simulink model "ammclib_gflib_limit_s32k14x"  (Simulink 9.0)
settings: Solver=FixedStepDiscrete  StartTime=0.0  StopTime=5  FixedStep=0.001  RelTol=1e-3  EnableMultiTasking=on
InitFcn:
  | mbd_s32k_consistency_checks(bdroot(gcs));
undefined symbols (not defined in the file or in its folder): LQFP
libraries: ammclib_bam_s32k14x x23, simulink x16, mbd_s32k1xx_ec_toolbox x2
Description:
  | This model tests the AMMCLIB GFLIB LIMIT blocks
  | 
  | Validation:
  | - Run the model in Simulation and check the results
  | - Open Freemaster (ammclib_gflib_limit_s32k14x.pmp) and compare the HW results against the Simulated ones
CloseFcn:
  | clear all;
settings Model: Creator=NXP MBDT Team  LastModifiedBy=nxf35172
settings DataIOCC: ExternalInput=off  InitialState=off  LimitDataPoints=on  SaveOutput=off  SignalLogging=off  SaveTime=off
settings OptimizationCC: DefaultParameterBehavior=Inlined  LifeSpan=1
settings DebuggingCC: SolverPrmCheckMsg=warning  InheritedTsInSrcMsg=none  SingleTaskRateTransMsg=error  IntegerOverflowMsg=none  ParameterPrecisionLossMsg=none  UnconnectedInputMsg=error  UnconnectedOutputMsg=error  UnconnectedLineMsg=error  AllowSymbolicDim=off  UnknownTsInhSupMsg=error  StateNameClashWarn=warning
settings HardwareCC: ProdLargestAtomicInteger=Long  ProdLargestAtomicFloat=Double  ProdEndianess=LittleEndian  ProdHWDeviceType=ARM Compatible->ARM Cortex
settings SFSimCC: MATLABDynamicMemAlloc=off
settings RTWCC: SystemTargetFile=mbd_s32k.tlc  MakeCommand=mbd_s32k_make_rtw COPY_MDLREF_INCLUDES=0  TemplateMakefile=mbd_s32k.tmf  Description=Model Based Design Toolbox S32K14x Code Generation Target
settings CodeAppCC: IgnoreCustomStorageClasses=off
settings STFCustomTargetCC: CombineOutputUpdateFcns=on  ERTCustomFileBanners=on  SupportContinuousTime=off  SupportNonInlinedSFcns=off  RemoveResetFunc=on  MATLABClassNameForMDSCustomization=Simulink.SoftwareTarget.ERTCustomization  GRTInterface=off  SystemTargetFile=mbd_s32k14.tlc
settings ERTTargetCC: MultiwordLength=2048  ParMdlRefBuildCompliant=off  CompOptLevelCompliant=off  ConcurrentExecutionCompliant=off  ModelStepFunctionPrototypeControlCompliant=off  CPPClassGenCompliant=off  UseToolchainInfoCompliant=off  InlinedParameterPlacement=NonHierarchical  ERTCustomFileTemplate=example_file_process.tlc  ConvertIfToSwitch=off  SuppressUnreachableDefaultCases=off

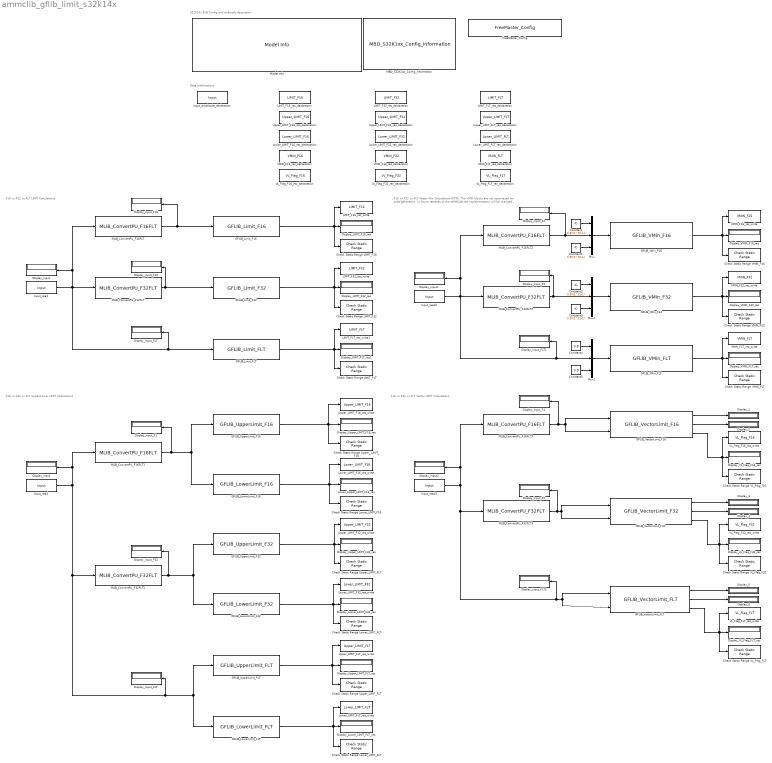
== system ammclib_gflib_limit_s32k14x ==
  note: S32K14x EVB Config and example description
  note: Data Initializations
  note: F16 vs F32 vs FLT LIMIT Calculations
  note: F16 vs F32 vs FLT Upper/Lower LIMIT Calculations
  note: F16 vs F32 vs FLT Vector Min Calculations
      | NOTE: The VMIN blocks are not optimiezed for code-generation. In future releases of the AMMCLIB the implementation will be changed
  note: F16 vs F32 vs FLT Vector LIMIT Calculations
  "Check Static Range LIMIT_F16 " : simulink/Model Verification/Check  Static Range  Description=-0.5*(2^15-1)-1 <= u <= 0.5*(2^15-1)+1  max=0.5*(2^15-1)+1  max_included=on  min=-0.5*(2^15-1)-1  min_included=on  enabled=on  stopWhenAssertionFail=on  export=off  icon=graphic
      settings: SourceProductName=Simulink  SourceProductBaseCode=SL
  Check Static Range LIMIT_F32 : simulink/Model Verification/Check  Static Range  Description=-0.5*(2^31-1)-1 <= u <= 0.5*(2^31-1)+1  max=0.5*(2^31-1)+1  max_included=on  min=-0.5*(2^31-1)-1  min_included=on  enabled=on  stopWhenAssertionFail=on  export=off  icon=graphic
      settings: SourceProductName=Simulink  SourceProductBaseCode=SL
  Check Static Range LIMIT_FLT : simulink/Model Verification/Check  Static Range  Description=-0.51 <= u <= 0.51  max=0.51  max_included=on  min=-0.51  min_included=on  enabled=on  stopWhenAssertionFail=on  export=off  icon=graphic
      settings: SourceProductName=Simulink  SourceProductBaseCode=SL
  Check Static Range Lower_LIMIT_F16 : simulink/Model Verification/Check  Static Range  Description=-0.5*(2^15-1)-1 <= u <= (2^15-1)  max=(2^15-1)  max_included=on  min=-0.5*(2^15-1)-1  min_included=on  enabled=on  stopWhenAssertionFail=on  export=off  icon=graphic
      settings: SourceProductName=Simulink  SourceProductBaseCode=SL
  Check Static Range Lower_LIMIT_FLT : simulink/Model Verification/Check  Static Range  Description=-0.5*(2^31-1)-1 <= u <= (2^31-1)  max=(2^31-1)  max_included=on  min=-0.5*(2^31-1)-1  min_included=on  enabled=on  stopWhenAssertionFail=on  export=off  icon=graphic
      settings: SourceProductName=Simulink  SourceProductBaseCode=SL
  "Check Static Range Lower_LIMIT_FLT  " : simulink/Model Verification/Check  Static Range  Description=-0.5 <= u <= 1  max=1  max_included=on  min=-0.5  min_included=on  enabled=on  stopWhenAssertionFail=on  export=off  icon=graphic
      settings: SourceProductName=Simulink  SourceProductBaseCode=SL
  "Check Static Range Upper_ LIMIT_F16 " : simulink/Model Verification/Check  Static Range  Description=-(2^15-1) <= u <= 0.5*(2^15-1)+1  max=0.5*(2^15-1)+1  max_included=on  min=-(2^15-1)  min_included=on  enabled=on  stopWhenAssertionFail=on  export=off  icon=graphic
      settings: SourceProductName=Simulink  SourceProductBaseCode=SL
  Check Static Range Upper_LIMIT_FLT : simulink/Model Verification/Check  Static Range  Description=-(2^31-1) <= u <= 0.5*(2^31-1)+1  max=0.5*(2^31-1)+1  max_included=on  min=-(2^31-1)  min_included=on  enabled=on  stopWhenAssertionFail=on  export=off  icon=graphic
      settings: SourceProductName=Simulink  SourceProductBaseCode=SL
  "Check Static Range Upper_LIMIT_FLT " : simulink/Model Verification/Check  Static Range  Description=-1 <= u <= 0.51  max=0.51  max_included=on  min=-1  min_included=on  enabled=on  stopWhenAssertionFail=on  export=off  icon=graphic
      settings: SourceProductName=Simulink  SourceProductBaseCode=SL
  Check Static Range VL_Flag_F32 : simulink/Model Verification/Check  Static Range  Description=0 <= u <= 1  max=1  max_included=on  min=0  min_included=on  enabled=on  stopWhenAssertionFail=on  export=off  icon=graphic
      settings: SourceProductName=Simulink  SourceProductBaseCode=SL
  Check Static Range VL_Flag_FLT : simulink/Model Verification/Check  Static Range  Description=0 <= u <= 1  max=1  max_included=on  min=0  min_included=on  enabled=on  stopWhenAssertionFail=on  export=off  icon=graphic
      settings: SourceProductName=Simulink  SourceProductBaseCode=SL
  Check Static Range VL_Flag_f16 : simulink/Model Verification/Check  Static Range  Description=0 <= u <= 1  max=1  max_included=on  min=0  min_included=on  enabled=on  stopWhenAssertionFail=on  export=off  icon=graphic
      settings: SourceProductName=Simulink  SourceProductBaseCode=SL
  Check Static Range VMIN_F16 : simulink/Model Verification/Check  Static Range  Description=0 <= u <= 2  max=2  max_included=on  min=0  min_included=on  enabled=on  stopWhenAssertionFail=on  export=off  icon=graphic
      settings: SourceProductName=Simulink  SourceProductBaseCode=SL
  Check Static Range VMIN_F32 : simulink/Model Verification/Check  Static Range  Description=0 <= u <= 2  max=2  max_included=on  min=0  min_included=on  enabled=on  stopWhenAssertionFail=on  export=off  icon=graphic
      settings: SourceProductName=Simulink  SourceProductBaseCode=SL
  Check Static Range VMIN_FLT : simulink/Model Verification/Check  Static Range  Description=0 <= u <= 2  max=2  max_included=on  min=0  min_included=on  enabled=on  stopWhenAssertionFail=on  export=off  icon=graphic
      settings: SourceProductName=Simulink  SourceProductBaseCode=SL
  Constant : Constant  Value=0.8*(2^15-1)  OutDataTypeStr=int16
  Constant1 : Constant  Value=0.9*(2^15-1)  OutDataTypeStr=int16
  Constant2 : Constant  Value=0.8*(2^31-1)  OutDataTypeStr=int32
  Constant3 : Constant  Value=0.9*(2^31-1)  OutDataTypeStr=int32
  Constant4 : Constant  Value=0.8  OutDataTypeStr=single
  Constant5 : Constant  Value=0.9  OutDataTypeStr=single
  Display_{1..6} (6 alike) : Display
  Display_LIMIT_F16_res : Display
  Display_LIMIT_F32_res : Display
  Display_LIMIT_FLT_res1 : Display
  Display_Lower_LIMIT_F32_res : Display
  Display_Lower_LIMIT_FLT_res : Display
  Display_Upper_LIMIT_F16_res : Display
  Display_Upper_LIMIT_F32_res : Display
  Display_Upper_LIMIT_FLT_res : Display
  Display_VL_Flag_F16_res : Display
  Display_VL_Flag_F32_res : Display
  Display_VL_Flag_FLT_res : Display
  Display_VMIN_F16_res : Display
  Display_VMIN_F32_res : Display
  Display_VMIN_FLT_res : Display
  Display_input : Display
  "Display_input  " : Display
  Display_input1 : Display
  Display_input2 : Display
  Display_input_F{1..5,16,32} (7 alike) : Display
  "Display_input_F32  " : Display
  Display_input_FLT : Display
  "Display_input_FLT  " : Display
  Display_input_FLT1 : Display
  Display_input_FLT2 : Display
  FreeMaster_Config : mbd_s32k1xx_ec_toolbox/Utility Blocks/FreeMaster_Config  interface=LPUART1  baudrate=115200  rxd=PTC6: [LPUART1_RX | Receive]  txd=PTC7: [LPUART1_TX | Transmit]  mode=Long Interrupt  isr_prio=1  show_adv_opts=on  use_scope=on  max_scope_vars=8  use_recorder=off  max_rec_vars=8  rec_buff_size=1024  rec_timebase=0 milliseconds  comm_buffer_size_auto=on  comm_buffer_size=255  comm_rqueue_size_default=on  comm_rqueue_size=32
  GFLIB_Limit_F16 : ammclib_bam_s32k14x/GFLIB/bam_f16/GFLIB_Limit_F16  f16UpperLimit=0.5*(2^15-1)  f16LowerLim=-0.5*(2^15-1)
  GFLIB_Limit_F32 : ammclib_bam_s32k14x/GFLIB/bam_f32/GFLIB_Limit_F32  f32UpperLimit=0.5*(2^31-1)  f32LowerLim=-0.5*(2^31-1)
  GFLIB_Limit_FLT : ammclib_bam_s32k14x/GFLIB/bam_flt/GFLIB_Limit_FLT  fltUpperLimit=0.5  fltLowerLim=-0.5
  GFLIB_LowerLimit_F16 : ammclib_bam_s32k14x/GFLIB/bam_f16/GFLIB_LowerLimit_F16  f16LowerLim=-0.5*(2^15-1)
  GFLIB_LowerLimit_F32 : ammclib_bam_s32k14x/GFLIB/bam_f32/GFLIB_LowerLimit_F32  f32LowerLim=-0.5*(2^31-1)
  GFLIB_LowerLimit_FLT : ammclib_bam_s32k14x/GFLIB/bam_flt/GFLIB_LowerLimit_FLT  fltLowerLim=-0.5
  GFLIB_UpperLimit_F16 : ammclib_bam_s32k14x/GFLIB/bam_f16/GFLIB_UpperLimit_F16  f16UpperLim=0.5*(2^15-1)
  GFLIB_UpperLimit_F32 : ammclib_bam_s32k14x/GFLIB/bam_f32/GFLIB_UpperLimit_F32  f32UpperLim=0.5*(2^31-1)
  GFLIB_UpperLimit_FLT : ammclib_bam_s32k14x/GFLIB/bam_flt/GFLIB_UpperLimit_FLT  fltUpperLim=0.5
  GFLIB_VMin_F16 : ammclib_bam_s32k14x/GFLIB/bam_f16/GFLIB_VMin_F16  N=3
  GFLIB_VMin_F32 : ammclib_bam_s32k14x/GFLIB/bam_f32/GFLIB_VMin_F32  N=3
  GFLIB_VMin_FLT : ammclib_bam_s32k14x/GFLIB/bam_flt/GFLIB_VMin_FLT  N=3
  GFLIB_VectorLimit_F16 : ammclib_bam_s32k14x/GFLIB/bam_f16/GFLIB_VectorLimit_F16  f16Limit=0.5*(2^15-1)
  GFLIB_VectorLimit_F32 : ammclib_bam_s32k14x/GFLIB/bam_f32/GFLIB_VectorLimit_F32  f32Limit=0.5*(2^31-1)
  GFLIB_VectorLimit_FLT : ammclib_bam_s32k14x/GFLIB/bam_flt/GFLIB_VectorLimit_FLT  fltLimit=0.5
  Input_Amplitude_declaration : DataStoreMemory  Priority=1  DataStoreName=Input  WriteAfterWriteMsg=warning  WriteAfterReadMsg=warning  InitialValue=0.75  ShowAdditionalParam=off  OutMin=-1  OutMax=1  OutDataTypeStr=single
  Input_read : DataStoreRead  DataStoreName=Input
  "Input_read  " : DataStoreRead  DataStoreName=Input
  Input_read1 : DataStoreRead  DataStoreName=Input
  Input_read2 : DataStoreRead  DataStoreName=Input
  LIMIT_F16_res_declaration : DataStoreMemory  Priority=2  DataStoreName=LIMIT_F16  ReadBeforeWriteMsg=warning  WriteAfterWriteMsg=warning  WriteAfterReadMsg=warning  ShowAdditionalParam=off  OutDataTypeStr=int16
  LIMIT_F16_res_write : DataStoreWrite  DataStoreName=LIMIT_F16
  LIMIT_F32_res_declaration : DataStoreMemory  Priority=2  DataStoreName=LIMIT_F32  ReadBeforeWriteMsg=warning  WriteAfterWriteMsg=warning  WriteAfterReadMsg=warning  ShowAdditionalParam=off  OutDataTypeStr=int32
  LIMIT_F32_res_write : DataStoreWrite  DataStoreName=LIMIT_F32
  LIMIT_FLT_res_declaration : DataStoreMemory  Priority=2  DataStoreName=LIMIT_FLT  ReadBeforeWriteMsg=warning  WriteAfterWriteMsg=warning  WriteAfterReadMsg=warning  ShowAdditionalParam=off  OutDataTypeStr=single
  LIMIT_FLT_res_write1 : DataStoreWrite  DataStoreName=LIMIT_FLT
  Lower_LIMIT_F16_res_declaration : DataStoreMemory  Priority=2  DataStoreName=Lower_LIMIT_F16  ReadBeforeWriteMsg=warning  WriteAfterWriteMsg=warning  WriteAfterReadMsg=warning  ShowAdditionalParam=off  OutDataTypeStr=int16
  Lower_LIMIT_F16_res_write : DataStoreWrite  DataStoreName=Lower_LIMIT_F16
  Lower_LIMIT_F32_res_declaration : DataStoreMemory  Priority=2  DataStoreName=Lower_LIMIT_F32  ReadBeforeWriteMsg=warning  WriteAfterWriteMsg=warning  WriteAfterReadMsg=warning  ShowAdditionalParam=off  OutDataTypeStr=int32
  Lower_LIMIT_F32_res_write : DataStoreWrite  DataStoreName=Lower_LIMIT_F32
  Lower_LIMIT_FLT_res_declaration : DataStoreMemory  Priority=2  DataStoreName=Lower_LIMIT_FLT  ReadBeforeWriteMsg=warning  WriteAfterWriteMsg=warning  WriteAfterReadMsg=warning  ShowAdditionalParam=off  OutDataTypeStr=single
  Lower_LIMIT_FLT_res_write : DataStoreWrite  DataStoreName=Lower_LIMIT_FLT
  Lower_Upper_LIMIT_F16_res : Display
  MBD_S32K14x_Config_Information : mbd_s32k1xx_ec_toolbox/MBD_S32K1xx_Config_Information  Priority=0  mbdt_ver=0  disp_str=|  config_params=[]  mcu_target_name=S32K144  mcu_target_package=100-LQFP  mcu_target_sram_size=64KB  mcu_system_clock_freq=80  mcu_xtal_freq=External 8  mcu_steptick_timer=LPIT Channel 0  mcu_steptick_prio=15  ds_import_enable=on  target_compiler=GCC  target_memory=FLASH  gcc_target_compile_opts=-mcpu=cortex-m4 -mthumb -mfloat-abi=hard -mfpu=fpv4-sp-d16 -O1 -g -gstrict-dwarf  gcc_target_assemble_opts=-mcpu=cortex-m4 -mthumb -mfloat-abi=hard -mfpu=fpv4-sp-d16 -g  gcc_target_link_opts=-mcpu=cortex-m4 -mthumb -mfloat-abi=hard -mfpu=fpv4-sp-d16  gcc_target_default_lcf=on  gcc_target_user_lcf=S32K144_64_flash.ld  ghs_target_compile_opts=-cpu=cortexm4f -thumb -DARM_MATH_CM4 -fpu=vfpv4_d16 -fsingle -Ogeneral -Wundef -Wimplicit-int -Wshadow -Wtrigraphs --no_commons --gnu_asm -gnu99 -gdwarf-2 -G  ghs_target_assemble_opts=-cpu=cortexm4f -fpu=vfpv4_d16  ghs_target_link_opts=-cpu=cortexm4f -thumb -fpu=vfpv4_d16  ghs_target_default_lcf=off  ghs_target_user_lcf=S32K144_64_flash.ld  iar_target_compile_opts=--cpu=Cortex-M4F --thumb --fpu=VFPv4_sp -Ol -e --debug --dlib_config normal  iar_target_assemble_opts=--cpu Cortex-M4F --thumb --fpu VFPv4_sp  iar_target_link_opts=--no_exceptions --vfe --inline  iar_target_default_lcf=off  iar_target_user_lcf=S32K144_64_flash.icf  pil_download_enable=off  rbl_download_enable=on  rbl_start_delay=5000000  rbl_download_interface=OpenSDA  rbl_restart_request=off  rbl_com_port=Custom  rbl_com_port_custom=COM1  pil_download_rate=57600  pil_opensda_drive=Custom  pil_opensda_drive_custom=D  pil_uart_instance=0  pil_uart_rx=PTA2: [LPUART0_RX | Receive]  pil_uart_tx=PTA3: [LPUART0_TX | Transmit]  FTM_PWM_PcrCheckEnDis=on  FTM_Input_Edge_Inputs_PcrCheckEnDis=on  FTM_Dual_Edge_Inputs_PcrCheckEnDis=on  FTM_Quadrature_Inputs_PcrCheckEnDis=on  FTM_Hall_Sensor_Inputs_PcrCheckEnDis=on  LPTMR_PcrCheckEnDis=on  PIT_PcrCheckEnDis=on  RTC_PcrCheckEnDis=on  FlexCAN_PcrCheckEnDis=on  LIN_PcrCheckEnDis=on  FlexIO_PcrCheckEnDis=on  LPI2C_PcrCheckEnDis=on  LPSPI_PcrCheckEnDis=on  LPUART_PcrCheckEnDis=on  CMP_PcrCheckEnDis=on  GPIO_OutputPcrCheckEnDis=on  GPIO_InputPcrCheckEnDis=on  SBC_PcrCheckEnDis=on  AMMCLIB_PcrCheckEnDis=on  FM_PcrCheckEnDis=on  Profile_PcrCheckEnDis=on  ConfigParams_PcrCheckEnDis=on  ModelRef_PcrCheckEnDis=on  PDB0_PcrCheckEnDis=on  CSEc_PcrCheckEnDis=on  eDMA_PcrCheckEnDis=on  ADC_PcrCheckEnDis=on  WDOG_PcrCheckEnDis=on
      | Target : S32K142-16KB_SRAM
      | Package : 100-pin
      | System clock : 80 MHz
      | XTAL clock : External 8 MHz
      | Compiler : GCC
      | Target Type : FLASH
      | Download Code after build : (OpenSDA: E)
      | Step Tick Interrupt Priority : 15
  MLIB_ConvertPU_F16FLT{,1..3} (4 alike) : ammclib_bam_s32k14x/MLIB/bam_f16/MLIB_ConvertPU_F16FLT
  MLIB_ConvertPU_F32FLT{,1..3} (4 alike) : ammclib_bam_s32k14x/MLIB/bam_f32/MLIB_ConvertPU_F32FLT
  Model Info : simulink/Model-Wide Utilities/Model Info  Frame=off  DisplayStringWithTags=|  HorizontalTextAlignment=Left  LeftAlignmentValue=0.02
      | Model Name: %<ModelName>
      | 
      | Description: %<Description>
  Mux : Mux  Inputs=3
  Mux1 : Mux  Inputs=3
  Mux2 : Mux  Inputs=3
  Upper_LIMIT_F16_res_declaration : DataStoreMemory  Priority=2  DataStoreName=Upper_LIMIT_F16  ReadBeforeWriteMsg=warning  WriteAfterWriteMsg=warning  WriteAfterReadMsg=warning  ShowAdditionalParam=off  OutDataTypeStr=int16
  Upper_LIMIT_F16_res_write : DataStoreWrite  DataStoreName=Upper_LIMIT_F16
  Upper_LIMIT_F32_res_declaration : DataStoreMemory  Priority=2  DataStoreName=Upper_LIMIT_F32  ReadBeforeWriteMsg=warning  WriteAfterWriteMsg=warning  WriteAfterReadMsg=warning  ShowAdditionalParam=off  OutDataTypeStr=int32
  Upper_LIMIT_F32_res_write : DataStoreWrite  DataStoreName=Upper_LIMIT_F32
  Upper_LIMIT_FLT_res_declaration : DataStoreMemory  Priority=2  DataStoreName=Upper_LIMIT_FLT  ReadBeforeWriteMsg=warning  WriteAfterWriteMsg=warning  WriteAfterReadMsg=warning  ShowAdditionalParam=off  OutDataTypeStr=single
  Upper_LIMIT_FLT_res_write : DataStoreWrite  DataStoreName=Upper_LIMIT_FLT
  VL_Flag_F16_res_declaration : DataStoreMemory  Priority=2  DataStoreName=VL_Flag_F16  ReadBeforeWriteMsg=warning  WriteAfterWriteMsg=warning  WriteAfterReadMsg=warning  ShowAdditionalParam=off  OutDataTypeStr=boolean
  VL_Flag_F16_res_write : DataStoreWrite  DataStoreName=VL_Flag_F16
  VL_Flag_F32_res_declaration : DataStoreMemory  Priority=2  DataStoreName=VL_Flag_F32  ReadBeforeWriteMsg=warning  WriteAfterWriteMsg=warning  WriteAfterReadMsg=warning  ShowAdditionalParam=off  OutDataTypeStr=boolean
  VL_Flag_F32_res_write : DataStoreWrite  DataStoreName=VL_Flag_F32
  VL_Flag_FLT_res_declaration : DataStoreMemory  Priority=2  DataStoreName=VL_Flag_FLT  ReadBeforeWriteMsg=warning  WriteAfterWriteMsg=warning  WriteAfterReadMsg=warning  ShowAdditionalParam=off  OutDataTypeStr=boolean
  VL_Flag_FLT_res_write : DataStoreWrite  DataStoreName=VL_Flag_FLT
  VMIN_F16_res_declaration : DataStoreMemory  Priority=2  DataStoreName=VMIN_F16  ReadBeforeWriteMsg=warning  WriteAfterWriteMsg=warning  WriteAfterReadMsg=warning  ShowAdditionalParam=off  OutDataTypeStr=uint16
  VMIN_F16_res_write : DataStoreWrite  DataStoreName=VMIN_F16
  VMIN_F32_res_declaration : DataStoreMemory  Priority=2  DataStoreName=VMIN_F32  ReadBeforeWriteMsg=warning  WriteAfterWriteMsg=warning  WriteAfterReadMsg=warning  ShowAdditionalParam=off  OutDataTypeStr=uint32
  VMIN_F32_res_write : DataStoreWrite  DataStoreName=VMIN_F32
  VMIN_FLT_res_declaration : DataStoreMemory  Priority=2  DataStoreName=VMIN_FLT  ReadBeforeWriteMsg=warning  WriteAfterWriteMsg=warning  WriteAfterReadMsg=warning  ShowAdditionalParam=off  OutDataTypeStr=uint32
  VMIN_FLT_res_write : DataStoreWrite  DataStoreName=VMIN_FLT
  wires:
  Input_read/1 -> Display_input_FLT/1, GFLIB_Limit_FLT/1, MLIB_ConvertPU_F16FLT/1, Display_input/1, MLIB_ConvertPU_F32FLT/1
  MLIB_ConvertPU_F16FLT/1 -> Display_input_F16/1, GFLIB_Limit_F16/1
  GFLIB_Limit_F16/1 -> LIMIT_F16_res_write/1, Display_LIMIT_F16_res/1, "Check Static Range LIMIT_F16 "/1
  MLIB_ConvertPU_F32FLT/1 -> GFLIB_Limit_F32/1, Display_input_F32/1
  GFLIB_Limit_F32/1 -> Check Static Range LIMIT_F32/1, LIMIT_F32_res_write/1, Display_LIMIT_F32_res/1
  GFLIB_Limit_FLT/1 -> Display_LIMIT_FLT_res1/1, LIMIT_FLT_res_write1/1, Check Static Range LIMIT_FLT/1
  "Input_read  "/1 -> "Display_input_FLT  "/1, GFLIB_UpperLimit_FLT/1, GFLIB_LowerLimit_FLT/1, MLIB_ConvertPU_F32FLT1/1, MLIB_ConvertPU_F16FLT1/1, "Display_input  "/1
  MLIB_ConvertPU_F16FLT1/1 -> GFLIB_LowerLimit_F16/1, GFLIB_UpperLimit_F16/1, Display_input_F1/1
  GFLIB_UpperLimit_F16/1 -> Upper_LIMIT_F16_res_write/1, Display_Upper_LIMIT_F16_res/1, "Check Static Range Upper_ LIMIT_F16 "/1
  MLIB_ConvertPU_F32FLT1/1 -> GFLIB_UpperLimit_F32/1, GFLIB_LowerLimit_F32/1, "Display_input_F32  "/1
  GFLIB_UpperLimit_F32/1 -> Check Static Range Upper_LIMIT_FLT/1, Upper_LIMIT_F32_res_write/1, Display_Upper_LIMIT_F32_res/1
  GFLIB_UpperLimit_FLT/1 -> Display_Upper_LIMIT_FLT_res/1, Upper_LIMIT_FLT_res_write/1, "Check Static Range Upper_LIMIT_FLT "/1
  GFLIB_LowerLimit_F16/1 -> Check Static Range Lower_LIMIT_F16/1, Lower_LIMIT_F16_res_write/1, Lower_Upper_LIMIT_F16_res/1
  GFLIB_LowerLimit_F32/1 -> Check Static Range Lower_LIMIT_FLT/1, Lower_LIMIT_F32_res_write/1, Display_Lower_LIMIT_F32_res/1
  GFLIB_LowerLimit_FLT/1 -> "Check Static Range Lower_LIMIT_FLT  "/1, Lower_LIMIT_FLT_res_write/1, Display_Lower_LIMIT_FLT_res/1
  MLIB_ConvertPU_F16FLT2/1 -> Mux/2, Display_input_F2/1
  GFLIB_VMin_F16/1 -> Check Static Range VMIN_F16/1, VMIN_F16_res_write/1, Display_VMIN_F16_res/1
  GFLIB_VMin_F32/1 -> Check Static Range VMIN_F32/1, VMIN_F32_res_write/1, Display_VMIN_F32_res/1
  GFLIB_VMin_FLT/1 -> Display_VMIN_FLT_res/1, VMIN_FLT_res_write/1, Check Static Range VMIN_FLT/1
  Mux/1 -> GFLIB_VMin_F16/1
  Constant/1 -> Mux/1
  Constant1/1 -> Mux/3
  MLIB_ConvertPU_F32FLT2/1 -> Mux1/2, Display_input_F3/1
  Mux1/1 -> GFLIB_VMin_F32/1
  Constant2/1 -> Mux1/1
  Constant3/1 -> Mux1/3
  Input_read1/1 -> Mux2/2, Display_input_FLT1/1, MLIB_ConvertPU_F16FLT2/1, Display_input1/1, MLIB_ConvertPU_F32FLT2/1
  Mux2/1 -> GFLIB_VMin_FLT/1
  Constant4/1 -> Mux2/1
  Constant5/1 -> Mux2/3
  Input_read2/1 -> Display_input_FLT2/1, GFLIB_VectorLimit_FLT/1, GFLIB_VectorLimit_FLT/2, MLIB_ConvertPU_F32FLT3/1, MLIB_ConvertPU_F16FLT3/1, Display_input2/1
  MLIB_ConvertPU_F16FLT3/1 -> GFLIB_VectorLimit_F16/1, GFLIB_VectorLimit_F16/2, Display_input_F4/1
  MLIB_ConvertPU_F32FLT3/1 -> GFLIB_VectorLimit_F32/1, GFLIB_VectorLimit_F32/2, Display_input_F5/1
  GFLIB_VectorLimit_F16/1 -> Display_1/1
  GFLIB_VectorLimit_F16/2 -> Display_2/1
  GFLIB_VectorLimit_F16/3 -> Check Static Range VL_Flag_f16/1, VL_Flag_F16_res_write/1, Display_VL_Flag_F16_res/1
  GFLIB_VectorLimit_F32/1 -> Display_3/1
  GFLIB_VectorLimit_F32/2 -> Display_4/1
  GFLIB_VectorLimit_F32/3 -> Check Static Range VL_Flag_F32/1, Display_VL_Flag_F32_res/1, VL_Flag_F32_res_write/1
  GFLIB_VectorLimit_FLT/1 -> Display_5/1
  GFLIB_VectorLimit_FLT/2 -> Display_6/1
  GFLIB_VectorLimit_FLT/3 -> Check Static Range VL_Flag_FLT/1, VL_Flag_FLT_res_write/1, Display_VL_Flag_FLT_res/1
